simulink model "tres_dummy_random"  (Simulink 8.3)
settings: Solver=VariableStepDiscrete  StartTime=0.0  StopTime=65  RelTol=1e-3
libraries: tres_simulink_blockset x3
settings Model: Creator=matteo  LastModifiedBy=matteo
settings OptimizationCC: ExpressionDepthLimit=2147483647
settings DebuggingCC: FcnCallInpInsideContextMsg=EnableAllAsWarning
settings GRTTargetCC: CombineOutputUpdateFcns=on  GRTInterface=off

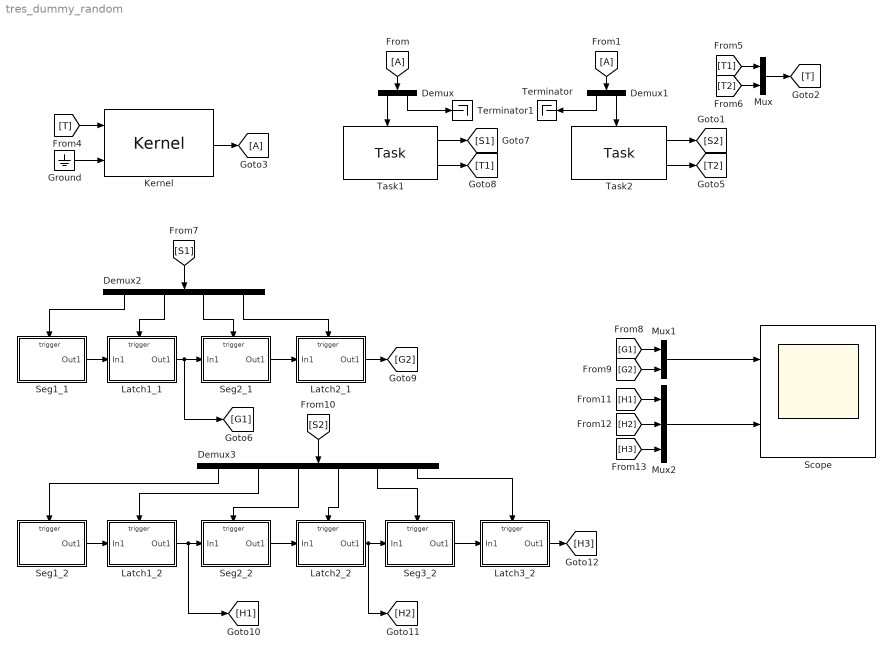
== system tres_dummy_random ==
  Demux : Demux  Outputs=2
  Demux1 : Demux  Outputs=2
  Demux2 : Demux
  Demux3 : Demux  Outputs=6
  Ground : Ground
  Kernel : tres_simulink_blockset/Kernel  taskset_descr_name=task_set_descr  scheduling_policy=DEADLINE_MONOTONIC  dead_miss_rule=Continue  time_res=Milli_Seconds  core_num=1  under_engine=RTSIM
  Latch1_1 : Subsystem  TreatAsAtomicUnit=on
  Latch1_2 : Subsystem  TreatAsAtomicUnit=on
  Latch2_1 : Subsystem  TreatAsAtomicUnit=on
  Latch2_2 : Subsystem  TreatAsAtomicUnit=on
  Latch3_2 : Subsystem  TreatAsAtomicUnit=on
  Mux : Mux  Inputs=2
  Mux1 : Mux  Inputs=2
  Mux2 : Mux  Inputs=3
  Scope : Scope  NumInputPorts=2
      settings: YMin=-5~-5  YMax=5~5
  Seg1_1 : Subsystem  TreatAsAtomicUnit=on
  Seg1_2 : Subsystem  TreatAsAtomicUnit=on
  Seg2_1 : Subsystem  TreatAsAtomicUnit=on
  Seg2_2 : Subsystem  TreatAsAtomicUnit=on
  Seg3_2 : Subsystem  TreatAsAtomicUnit=on
  Task1 : tres_simulink_blockset/Task  conf_name=t1_instrs
  Task2 : tres_simulink_blockset/Task  conf_name=t2_instrs
  Terminator : Terminator
  Terminator1 : Terminator
  wires:
  [A] -> Demux/1
  [A] -> Demux1/1
  [T] -> Kernel/1
  [T1] -> Mux/1
  [T2] -> Mux/2
  Mux/1 -> [T]
  Kernel/1 -> [A]
  Demux/1 -> Task1/Trigger
  Demux/2 -> Terminator1/1
  Demux1/2 -> Task2/Trigger
  Demux1/1 -> Terminator/1
  Task2/2 -> [T2]
  Task2/1 -> [S2]
  Task1/2 -> [T1]
  Task1/1 -> [S1]
  Seg1_1/1(Out1) -> Latch1_1/1(In1)
  Latch1_1/1(Out1) -> Seg2_1/1(In1), [G1]
  Seg2_1/1(Out1) -> Latch2_1/1(In1)
  Latch2_1/1(Out1) -> [G2]
  Demux2/1 -> Seg1_1/Trigger
  [S1] -> Demux2/1
  Demux2/2 -> Latch1_1/Trigger
  Demux2/3 -> Seg2_1/Trigger
  Demux2/4 -> Latch2_1/Trigger
  [G1] -> Mux1/1
  [G2] -> Mux1/2
  Mux1/1 -> Scope/1
  Seg1_2/1(Out1) -> Latch1_2/1(In1)
  Seg2_2/1(Out1) -> Latch2_2/1(In1)
  Latch2_2/1(Out1) -> [H2], Seg3_2/1(In1)
  Demux3/1 -> Seg1_2/Trigger
  [S2] -> Demux3/1
  Demux3/2 -> Latch1_2/Trigger
  Demux3/3 -> Seg2_2/Trigger
  Demux3/4 -> Latch2_2/Trigger
  [H1] -> Mux2/1
  [H2] -> Mux2/2
  Latch1_2/1(Out1) -> [H1], Seg2_2/1(In1)
  Seg3_2/1(Out1) -> Latch3_2/1(In1)
  Latch3_2/1(Out1) -> [H3]
  Demux3/5 -> Seg3_2/Trigger
  Demux3/6 -> Latch3_2/Trigger
  [H3] -> Mux2/3
  Mux2/1 -> Scope/2
  Ground/1 -> Kernel/2

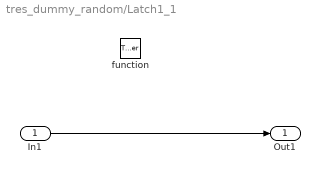
== system tres_dummy_random/Latch1_1 ==
  In1 : Inport
  function : TriggerPort  TriggerType=function-call
  Out1 : Outport
  wires:
  In1/1 -> Out1/1

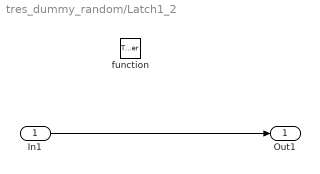
== system tres_dummy_random/Latch1_2 ==
  In1 : Inport
  function : TriggerPort  TriggerType=function-call
  Out1 : Outport
  wires:
  In1/1 -> Out1/1

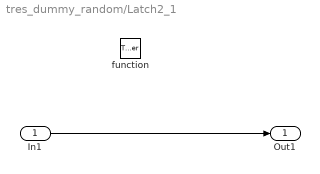
== system tres_dummy_random/Latch2_1 ==
  In1 : Inport
  function : TriggerPort  TriggerType=function-call
  Out1 : Outport
  wires:
  In1/1 -> Out1/1

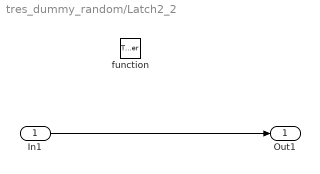
== system tres_dummy_random/Latch2_2 ==
  In1 : Inport
  function : TriggerPort  TriggerType=function-call
  Out1 : Outport
  wires:
  In1/1 -> Out1/1

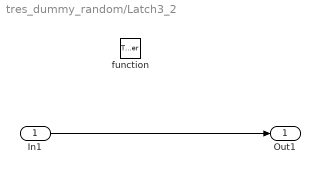
== system tres_dummy_random/Latch3_2 ==
  In1 : Inport
  function : TriggerPort  TriggerType=function-call
  Out1 : Outport
  wires:
  In1/1 -> Out1/1

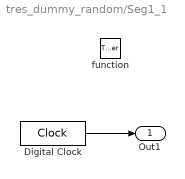
== system tres_dummy_random/Seg1_1 ==
  function : TriggerPort  TriggerType=function-call
  Digital Clock : DigitalClock  SampleTime=-1
  Out1 : Outport
  wires:
  Digital Clock/1 -> Out1/1

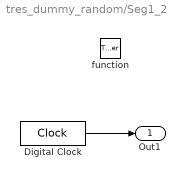
== system tres_dummy_random/Seg1_2 ==
  function : TriggerPort  TriggerType=function-call
  Digital Clock : DigitalClock  SampleTime=-1
  Out1 : Outport
  wires:
  Digital Clock/1 -> Out1/1

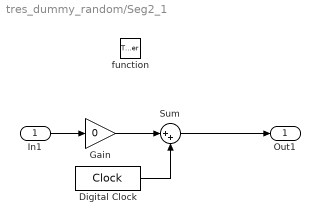
== system tres_dummy_random/Seg2_1 ==
  In1 : Inport
  function : TriggerPort  TriggerType=function-call
  Digital Clock : DigitalClock  SampleTime=-1
  Gain : Gain  Gain=0
  Sum : Sum  Inputs=|++
  Out1 : Outport
  wires:
  Sum/1 -> Out1/1
  Digital Clock/1 -> Sum/2
  In1/1 -> Gain/1
  Gain/1 -> Sum/1

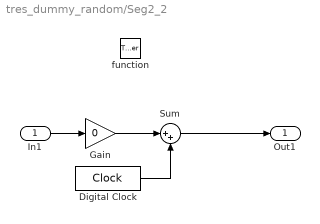
== system tres_dummy_random/Seg2_2 ==
  In1 : Inport
  function : TriggerPort  TriggerType=function-call
  Digital Clock : DigitalClock  SampleTime=-1
  Gain : Gain  Gain=0
  Sum : Sum  Inputs=|++
  Out1 : Outport
  wires:
  Sum/1 -> Out1/1
  Digital Clock/1 -> Sum/2
  In1/1 -> Gain/1
  Gain/1 -> Sum/1

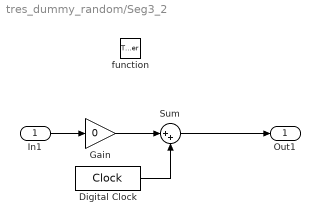
== system tres_dummy_random/Seg3_2 ==
  In1 : Inport
  function : TriggerPort  TriggerType=function-call
  Digital Clock : DigitalClock  SampleTime=-1
  Gain : Gain  Gain=0
  Sum : Sum  Inputs=|++
  Out1 : Outport
  wires:
  Sum/1 -> Out1/1
  Digital Clock/1 -> Sum/2
  In1/1 -> Gain/1
  Gain/1 -> Sum/1
